simulink model "hw7_q3_c"  (R2020b)
settings: Solver=FixedStepDiscrete  StartTime=0.0  StopTime=10.0  FixedStep=1/44100  RelTol=1e-3  EnableMultiTasking=on
model workspace (MATLAB code in the model file + MAT data in the model file):
  cmdLim = Simulink.Parameter
  cmdLim.Value = 15
  cmdLim.Description = 'Limit for controlling the maximum surface command angle.'
  cmdLim.Min = 0
  cmdLim.Max = 90
  cmdLim.DocUnits = 'deg'
  dispGain = Simulink.Parameter
  dispGain.Value = 0.75
  dispGain.Description = 'Gain applied to the displacement error.'
  dispGain.Min = 0
  dispGain.Max = []
  dispGain.DocUnits = 'deg/sec/deg'
  dispLim = Simulink.Parameter
  dispLim.Value = 30
  dispLim.Description = 'Limit for controlling the maximum commanded angle.'
  dispLim.Min = 0
  dispLim.Max = 180
  dispLim.DocUnits = 'deg'
  intGain = Simulink.Parameter
  intGain.Value = 0.5
  intGain.Description = 'Gain applied to the integral error.'
  intGain.Min = 0
  intGain.Max = []
  intGain.DocUnits = 'deg/sec/deg/sec'
  intLim = Simulink.Parameter
  intLim.Value = 5
  intLim.Description = 'Limit for controlling the maximum commanded angle.'
  intLim.Min = 0
  intLim.Max = 90
  intLim.DocUnits = 'deg'
  rateGain = Simulink.Parameter
  rateGain.Value = 2
  rateGain.Description = 'Gain applied to the rate error.'
  rateGain.Min = 0
  rateGain.Max = []
  rateGain.DocUnits = 'deg/deg/sec'
  rateLim = Simulink.Parameter
  rateLim.Value = 6
  rateLim.Description = 'Limit for controlling the maximum commanded angle.'
  rateLim.Min = 0
  rateLim.Max = 180
  rateLim.DocUnits = 'deg/sec'
  hdgGain = Simulink.Parameter
  hdgGain.Value = 0.015
  a = Simulink.Parameter
  a.Value = [-3.25656931096 4.03376839272 -2.24604368203 0.473506452939]
  a.DataType = 'auto'
  a.Dimensions = [1 4]
  b = Simulink.Parameter
  b.Value = [4 6 4 1]
  b.DataType = 'auto'
  b.Dimensions = [1 4]
  k = 0.00029137
settings Model: RequirementInfo={} %GIDa_fe9045fd_0412_4b6e_8206_617cc20e6fde  FPTRunName=Active  SILPILModeSetting=veronly  ExtModeTrigDuration=2  OrderedModelArguments=off  Creator=Hosein  LastModifiedBy=Hosein
settings SolverCC: AutoInsertRateTranBlk=on
settings DataIOCC: SaveOutput=off  SignalLogging=off  DSMLogging=off  SaveTime=off
settings OptimizationCC: UseDivisionForNetSlopeComputation=on  GainParamInheritBuiltInType=on  UseFloatMulNetSlope=on  UseSpecifiedMinMax=on  EnhancedBackFolding=on  PassReuseOutputArgsAs=Individual arguments  ZeroExternalMemoryAtStartup=off  ZeroInternalMemoryAtStartup=off  NoFixptDivByZeroProtection=on  EfficientFloat2IntCast=on  LifeSpan=1  MaxStackSize=64  OptimizeBlockOrder=speed  DifferentSizesBufferReuse=on  OptimizationCustomize=off  EfficientTunableParamExpr=on
settings DebuggingCC: AllowSymbolicDim=off  SFUnexpectedBacktrackingDiag=warning  SFNoUnconditionalDefaultTransitionDiag=warning  SFExecutionAtInitializationDiag=none  ArithmeticOperatorsInVariantConditions=warning
settings HardwareCC: ProdBitPerInt=16  ProdBitPerPointer=16  ProdBitPerSizeT=16  ProdBitPerPtrDiffT=16  ProdLargestAtomicFloat=None  ProdWordSize=8  ProdHWDeviceType=Atmel->AVR
settings SFSimCC: MATLABDynamicMemAlloc=off
settings RTWCC: Description=Embedded Coder  SystemTargetFile=ert.tlc  HardwareBoard=Arduino Mega 2560  GenCodeOnly=on  TemplateMakefile=ert_default_tmf  Toolchain=Arduino AVR  BuildConfiguration=Specify
settings CodeAppCC: ForceParamTrailComments=on  IgnoreCustomStorageClasses=off  OperatorAnnotations=on  SimulinkDataObjDesc=on  SFDataObjDesc=on  CustomSymbolStrGlobalVar=rt$N$M  CustomSymbolStrType=$N$M  CustomSymbolStrFcn=$N$M$F  CustomSymbolStrMacro=$N$M  InsertBlockDesc=on  EnableCustomComments=on  ReqsInCode=on
settings ERTTargetCC: UtilityFuncGeneration=Shared location  MultiwordLength=2048  CombineSignalStateStructs=on  SuppressErrorStatus=on  SupportNonFinite=off  SupportComplex=off  SupportContinuousTime=on  SupportVariableSizeSignals=on  ExtModeStaticAllocSize=2048  ERTFilePackagingFormat=CompactWithDataFile
settings ConfigComp: CovScope=ReferencedModels  CovSaveName=covdata_rollAP  CovMetricSettings=dcmtrwe  CovHTMLOptions=-sRT=1 -aTS=1 -bRG=1 -bTC=1 -hTR=1 -nFC=0 -scm=1 -bcm=1 -xEv=0  CovSaveCumulativeToWorkspaceVar=on  CovSaveSingleToWorkspaceVar=on  CovCumulativeVarName=covCumulativeData_rollAP  CovReportOnPause=off  CovExternalEMLEnable=off  CovSFcnEnable=off

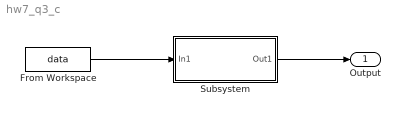
== system hw7_q3_c ==
  From Workspace : FromWorkspace  VariableName=data  SampleTime=1/44100
  Subsystem : Subsystem
  Output : Outport
  wires:
  From Workspace/1 -> Subsystem/1(In1)
  Subsystem/1(Out1) -> Output/1

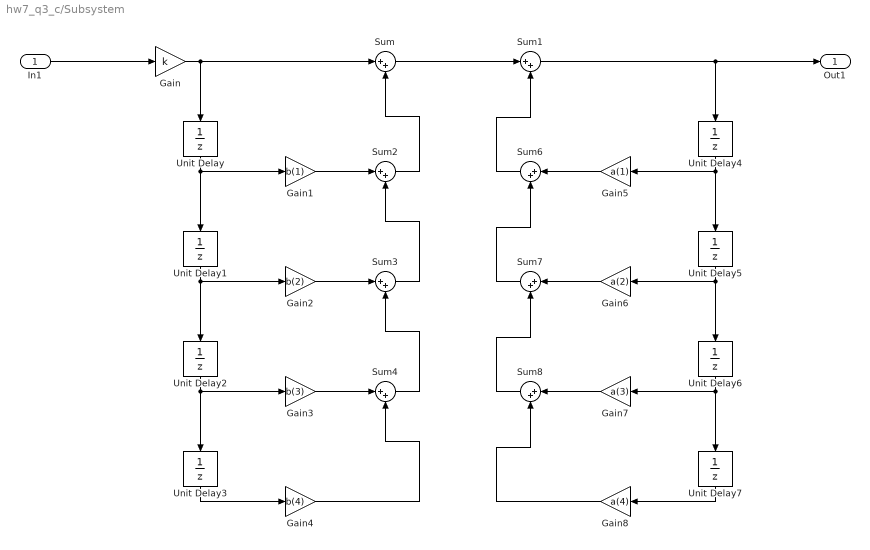
== system hw7_q3_c/Subsystem ==
  In1 : Inport
  Gain : Gain  Gain=k
  Gain1 : Gain  Gain=b(1)
  Gain2 : Gain  Gain=b(2)
  Gain3 : Gain  Gain=b(3)
  Gain4 : Gain  Gain=b(4)
  Gain5 : Gain  Gain=a(1)
  Gain6 : Gain  Gain=a(2)
  Gain7 : Gain  Gain=a(3)
  Gain8 : Gain  Gain=a(4)
  Sum{,1..4,6..8} (8 alike) : Sum  Inputs=|++
  Unit Delay{,1..7} (8 alike) : UnitDelay  SampleTime=-1  HasFrameUpgradeWarning=on
  Out1 : Outport
  wires:
  Gain8/1 -> Sum8/2
  Unit Delay7/1 -> Gain8/1
  Gain/1 -> Unit Delay/1, Sum/1
  Unit Delay5/1 -> Gain6/1, Unit Delay6/1
  Unit Delay6/1 -> Gain7/1, Unit Delay7/1
  Gain7/1 -> Sum8/1
  Unit Delay/1 -> Unit Delay1/1, Gain1/1
  Sum7/1 -> Sum6/2
  Unit Delay2/1 -> Unit Delay3/1, Gain3/1
  Gain6/1 -> Sum7/1
  Sum8/1 -> Sum7/2
  Unit Delay4/1 -> Gain5/1, Unit Delay5/1
  Gain5/1 -> Sum6/1
  Sum2/1 -> Sum/2
  Sum6/1 -> Sum1/2
  Unit Delay3/1 -> Gain4/1
  Unit Delay1/1 -> Unit Delay2/1, Gain2/1
  Gain4/1 -> Sum4/2
  Gain1/1 -> Sum2/1
  Gain3/1 -> Sum4/1
  Sum1/1 -> Out1/1, Unit Delay4/1
  Gain2/1 -> Sum3/1
  Sum3/1 -> Sum2/2
  Sum4/1 -> Sum3/2
  Sum/1 -> Sum1/1
  In1/1 -> Gain/1
